simulink model "gm_sampleModel1881_2_sub_sub"  (R2023a)
settings: Solver=VariableStepAuto  StartTime=0.0  StopTime=10.0  RelTol=1e-3
libraries: simulink x2, hdlsllib x2
settings Model: Creator=user1  LastModifiedBy=user1
settings OptimizationCC: BlockReduction=off  ConditionallyExecuteInputs=off
settings DebuggingCC: InheritedTsInSrcMsg=none

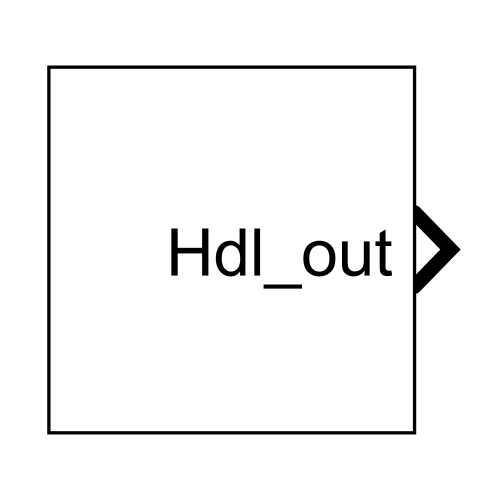
[thumbnail: Simulink's stored preview of the top-level diagram]
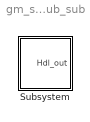
== system gm_sampleModel1881_2_sub_sub ==
  Subsystem : Subsystem

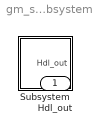
== system gm_sampleModel1881_2_sub_sub/Subsystem ==
  Subsystem : Subsystem
  Hdl_out : Outport  OutDataTypeStr=uint8

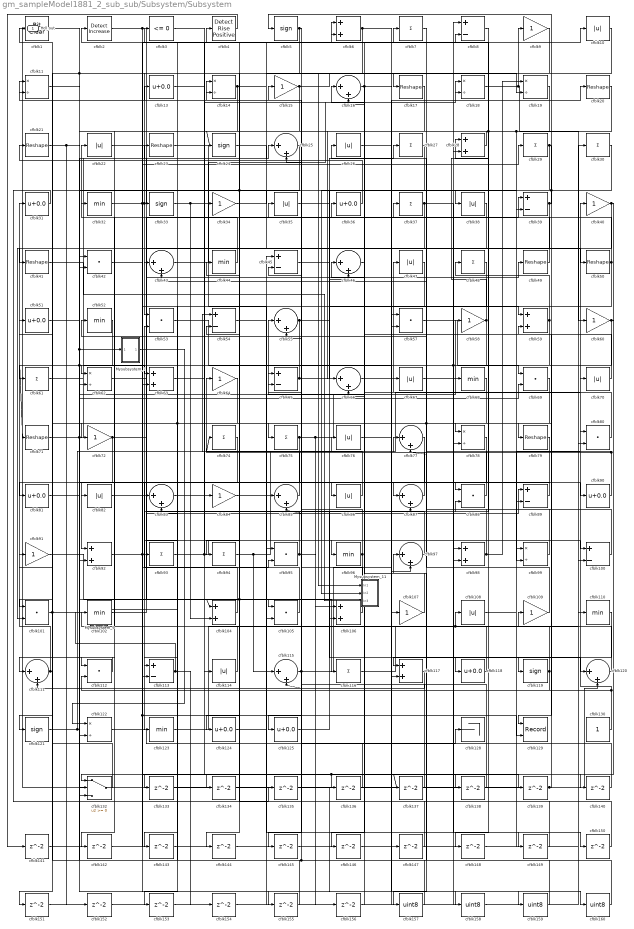
== system gm_sampleModel1881_2_sub_sub/Subsystem/Subsystem ==
  Mysubsystem_11 : Subsystem  TreatAsAtomicUnit=on  RTWFcnName=Mysubsystem_11
      settings: RTWFcnNameOpts=User specified  RTWFileNameOpts=Use function name
  Mysubsystem_7 : Subsystem  TreatAsAtomicUnit=on  RTWFcnName=Mysubsystem_7
      settings: RTWFcnNameOpts=User specified  RTWFileNameOpts=Use function name
  Mysubsystem_9 : Subsystem  TreatAsAtomicUnit=on  RTWFcnName=Mysubsystem_9
      settings: RTWFcnNameOpts=User specified  RTWFileNameOpts=Use function name
  cfblk1 : simulink/Logic and Bit Operations/Bit Clear  iBit=0
      settings: LibrarySourceBlock=|
      | hdlsllib/Logic and Bit
      | Operations/Bit Clear
  cfblk{10,22,26,35,38,47,67,70,76,82,86,108,114} (13 alike) : Abs  OutDataTypeStr=uint8  SaturateOnIntegerOverflow=off
  cfblk{8,39,45,54,65,89,100,113} (8 alike) : Sum  Inputs=+-  OutDataTypeStr=uint8
  cfblk{42,53,57,69,80,88,95,101,105,112} (10 alike) : DotProduct  OutDataTypeStr=uint8
  cfblk{32,44,52,68,96,102,110,123} (8 alike) : MinMax  OutDataTypeStr=uint8
  cfblk{6,28,59,63,92,98,104,106,117} (9 alike) : Sum  OutDataTypeStr=uint8
  cfblk{9,15,34,40,58,60,64,72,84,91,107,109} (12 alike) : Gain  OutDataTypeStr=uint8
  cfblk{11,14,18..19,62,78,99,122} (8 alike) : Product  Inputs=*/  OutDataTypeStr=uint8  RndMeth=Zero  SaturateOnIntegerOverflow=on
  cfblk{16,25,43,46,55,66,77,83,85,87,97,111,115,120} (14 alike) : Sum  Inputs=|++  OutDataTypeStr=uint8
  cfblk{7,27,29..30,37,48,61,74..75,93..94,116} (12 alike) : Sum  Inputs=+  OutDataTypeStr=uint8
  cfblk{13,31,36,51,81,90,118,124..125} (9 alike) : Bias  Bias=0.0  SaturateOnIntegerOverflow=off
  cfblk{5,24,33,119,121} (5 alike) : Signum
  cfblk128 : Terminator
  cfblk129 : Record  FileSettingsInternal="{\"entries\":[{\"content\":{\"excelSettings\":{\"content\":{},\"type\":\"Streamout.ExcelSettings\"}},\"type\":\"Streamout.FileSettingStorage\",\"uuid\":\"\"}],\"packageUris\":[\"http:\\/\\/schema.mathworks.com\\/mf0\\/streamout_blocks\\/R2020a\"],\"version\":\"1.0\"}"  Layout=[1 1]  SignalsInternal="{\"entries\":[{\"content\":{\"signals\":[{\"content\":{\"blockPath\":[],\"dimensions\":[1],\"domain\":\"\",\"lineColor\":\"#a2142f\",\"plots\":[1],\"port\":1,\"signalID\":47170,\"signalName\":\"cfblk29\"},\"type\":\"RecordBlkView.Signal\",\"uuid\":\"\"},{\"content\":{\"blockPath\":[],\"dimensions\":[1],\"domain\":\"\",\"lineColor\":\"#139fff\",\"plots\":[1],\"port\":2,\"signalID\":47173,\"signalName\":\"cfblk42\"},\"type\":\"RecordBlkView.Signal\",\"uuid\":\"\"}]},\"type\":\"RecordBlkView.InputSignals\",\"uuid\":\"\"}],\"packageUris\":[\"http:\\/\\/schema.mathworks.com\\/mf0\\/streamout_blocks\\/R2020a\"],\"version\":\"1.0\"}"  VisualizationBindings="{\"xyplotplugin\":{\"info\":[{\"series\":[{\"bindingParametersList\":[{\"parameter\":\"X-Axis\",\"signalID\":47170,\"signalName\":\"cfblk29\"},{\"parameter\":\"Y-Axis\",\"signalID\":47173,\"signalName\":\"cfblk42\"}],\"seriesID\":24383}],\"subplotID\":1}]}}"  CompatibilityTag=XY  st=-1
  cfblk130 : Constant  OutDataTypeStr=uint8  SampleTime=-1
  cfblk132 : Switch  OutDataTypeStr=uint8  SaturateOnIntegerOverflow=off  InputSameDT=off
  cfblk{133..156} (24 alike) : Delay  SampleTime=1
  cfblk{157..160} (4 alike) : DataTypeConversion  OutDataTypeStr=uint8  SaturateOnIntegerOverflow=off  RndMeth=Floor
  cfblk{17,20..21,23,41,49..50,71,79} (9 alike) : Reshape
  cfblk2 : simulink/Logic and Bit Operations/Detect Increase  vinit=0.0  OutDataTypeStr=uint8
      settings: LibrarySourceBlock=|
      | hdlsllib/Logic and Bit
      | Operations/Detect
      | Increase
  cfblk3 : hdlsllib/Logic and Bit Operations/Compare To Zero  relop=<=  OutDataTypeStr=uint8
  cfblk4 : hdlsllib/Logic and Bit Operations/Detect Rise Positive  vinit=0  OutDataTypeStr=uint8
  Hdl_out : Outport  OutDataTypeStr=uint8
  wires:
  cfblk88/1 -> cfblk26/1
  cfblk71/1 -> cfblk69/2, cfblk25/1
  cfblk93/1 -> cfblk10/1, cfblk96/1
  cfblk82/1 -> cfblk48/1
  cfblk86/1 -> cfblk64/1
  cfblk123/1 -> cfblk109/1
  cfblk28/1 -> cfblk66/1
  cfblk87/1 -> cfblk55/1
  cfblk130/1 -> cfblk15/1, cfblk40/1
  cfblk77/1 -> cfblk92/1
  cfblk121/1 -> cfblk76/1, cfblk54/1
  cfblk79/1 -> cfblk82/1
  cfblk58/1 -> cfblk125/1, cfblk2/1
  cfblk102/1 -> cfblk89/1
  cfblk80/1 -> cfblk35/1
  cfblk111/1 -> cfblk11/1, cfblk31/1
  cfblk110/1 -> cfblk157/1
  cfblk43/1 -> cfblk18/1
  cfblk19/1 -> cfblk24/1, cfblk118/1
  cfblk122/1 -> cfblk128/1
  cfblk37/1 -> cfblk150/1, cfblk94/1
  cfblk50/1 -> cfblk113/2, cfblk36/1
  cfblk57/1 -> cfblk69/1
  cfblk70/1 -> cfblk16/1
  cfblk47/1 -> cfblk75/1
  cfblk67/1 -> cfblk58/1
  cfblk94/1 -> cfblk115/1, cfblk70/1
  cfblk59/1 -> cfblk62/2, cfblk28/1
  cfblk34/1 -> cfblk38/1
  cfblk120/1 -> cfblk6/2, cfblk108/1
  cfblk75/1 -> cfblk133/1, cfblk156/1, cfblk57/2
  cfblk35/1 -> cfblk59/1
  cfblk78/1 -> cfblk123/1
  cfblk23/1 -> cfblk85/1
  cfblk2/1 -> cfblk155/1, cfblk100/1
  cfblk105/1 -> cfblk44/1
  cfblk95/1 -> cfblk106/1, cfblk14/1
  cfblk124/1 -> cfblk45/1
  cfblk39/1 -> cfblk99/2, cfblk5/1
  cfblk108/1 -> cfblk80/1
  cfblk8/1 -> cfblk78/1
  cfblk53/1 -> cfblk107/1
  cfblk62/1 -> cfblk39/1
  cfblk18/1 -> cfblk60/1, cfblk9/1
  cfblk66/1 -> cfblk47/1
  cfblk3/1 -> cfblk34/1
  cfblk63/1 -> cfblk18/2
  cfblk40/1 -> cfblk101/2, cfblk132/1
  cfblk92/1 -> cfblk95/2, cfblk29/1, cfblk49/1
  cfblk5/1 -> cfblk145/1, cfblk144/1
  cfblk36/1 -> cfblk21/1
  cfblk112/1 -> cfblk111/1
  cfblk30/1 -> cfblk106/2, cfblk79/1
  cfblk44/1 -> cfblk22/1
  cfblk118/1 -> cfblk3/1
  cfblk81/1 -> cfblk68/1
  cfblk91/1 -> cfblk105/1
  cfblk55/1 -> cfblk117/2, cfblk92/2, cfblk71/1
  cfblk109/1 -> cfblk67/1
  cfblk85/1 -> cfblk54/2
  cfblk14/1 -> cfblk19/2, cfblk72/1
  cfblk99/1 -> cfblk37/1
  cfblk60/1 -> cfblk140/1, cfblk98/2, cfblk105/2
  cfblk115/1 -> cfblk85/2, cfblk20/1
  cfblk98/1 -> cfblk19/1, cfblk77/1
  cfblk17/1 -> cfblk53/1
  cfblk107/1 -> cfblk46/1
  cfblk96/1 -> cfblk13/1, cfblk134/1, cfblk122/2
  cfblk38/1 -> cfblk121/1
  cfblk10/1 -> cfblk43/1
  cfblk20/1 -> cfblk148/1, cfblk89/2
  cfblk22/1 -> cfblk46/2
  cfblk119/1 -> cfblk112/2, cfblk102/1
  cfblk46/1 -> cfblk6/1
  cfblk49/1 -> cfblk4/1
  cfblk33/1 -> cfblk139/1, cfblk104/2
  cfblk25/1 -> cfblk81/1, cfblk124/1
  cfblk104/1 -> cfblk53/2
  cfblk100/1 -> cfblk52/1
  cfblk13/1 -> cfblk114/1
  cfblk29/1 -> cfblk86/1, cfblk129/1
  cfblk90/1 -> cfblk74/1, cfblk43/2
  cfblk51/1 -> cfblk90/1, Mysubsystem_7/1(In1)
  cfblk61/1 -> cfblk63/1
  cfblk74/1 -> cfblk113/1
  cfblk72/1 -> cfblk151/1, cfblk116/1
  cfblk11/1 -> cfblk132/2
  cfblk114/1 -> cfblk32/1
  cfblk84/1 -> cfblk87/1
  cfblk132/1 -> cfblk91/1
  cfblk97/1 -> cfblk83/1
  cfblk106/1 -> cfblk65/1, cfblk104/1
  cfblk101/1 -> cfblk51/1, cfblk23/1
  cfblk65/1 -> cfblk27/1, cfblk62/1
  cfblk83/1 -> cfblk84/1
  cfblk116/1 -> cfblk30/1
  cfblk15/1 -> cfblk17/1, cfblk132/3
  cfblk69/1 -> cfblk77/2, cfblk112/1, cfblk93/1
  cfblk21/1 -> cfblk152/1, cfblk39/2
  cfblk6/1 -> cfblk138/1, cfblk41/1, cfblk42/2
  cfblk24/1 -> cfblk50/1
  cfblk117/1 -> cfblk111/2
  cfblk7/1 -> cfblk117/1
  cfblk32/1 -> cfblk8/2, cfblk33/1, cfblk7/1
  cfblk42/1 -> cfblk129/2, cfblk137/1, cfblk136/1
  cfblk52/1 -> cfblk61/1
  cfblk89/1 -> cfblk88/1
  cfblk125/1 -> cfblk88/2
  cfblk16/1 -> cfblk146/1, cfblk119/1
  cfblk113/1 -> cfblk154/1, Mysubsystem_9/1(In1)
  cfblk45/1 -> cfblk120/1
  cfblk68/1 -> cfblk101/1
  cfblk133/1 -> cfblk28/2
  cfblk134/1 -> cfblk120/2
  cfblk31/1 -> cfblk135/1
  cfblk136/1 -> cfblk45/2
  cfblk137/1 -> cfblk11/2
  cfblk138/1 -> cfblk55/2
  cfblk139/1 -> Hdl_out/1, cfblk59/2
  cfblk140/1 -> cfblk25/2
  cfblk4/1 -> cfblk141/1
  cfblk141/1 -> cfblk63/2
  cfblk64/1 -> cfblk142/1
  cfblk142/1 -> cfblk98/1
  cfblk48/1 -> cfblk143/1
  cfblk143/1 -> cfblk57/1
  cfblk144/1 -> cfblk97/2
  cfblk145/1 -> cfblk65/2
  cfblk146/1 -> cfblk99/1
  cfblk26/1 -> cfblk147/1
  cfblk147/1 -> cfblk16/2
  cfblk148/1 -> cfblk80/2
  cfblk54/1 -> cfblk149/1
  cfblk149/1 -> cfblk14/2
  cfblk150/1 -> cfblk8/1
  cfblk151/1 -> cfblk95/1
  cfblk152/1 -> cfblk78/2
  cfblk153/1 -> cfblk100/2
  cfblk154/1 -> cfblk87/2
  cfblk155/1 -> cfblk83/2
  cfblk156/1 -> cfblk66/2
  cfblk157/1 -> cfblk42/1, cfblk115/2
  cfblk76/1 -> cfblk158/1
  cfblk158/1 -> cfblk110/1
  cfblk135/1 -> cfblk159/1
  cfblk159/1 -> cfblk1/1
  cfblk1/1 -> cfblk160/1
  cfblk160/1 -> cfblk97/1
  Mysubsystem_7/1(Out1) -> cfblk122/1
  Mysubsystem_9/1(Out1) -> cfblk153/1
  cfblk9/1 -> Mysubsystem_11/1(In1)
  cfblk27/1 -> Mysubsystem_11/2(In2)
  cfblk41/1 -> Mysubsystem_11/3(In3)

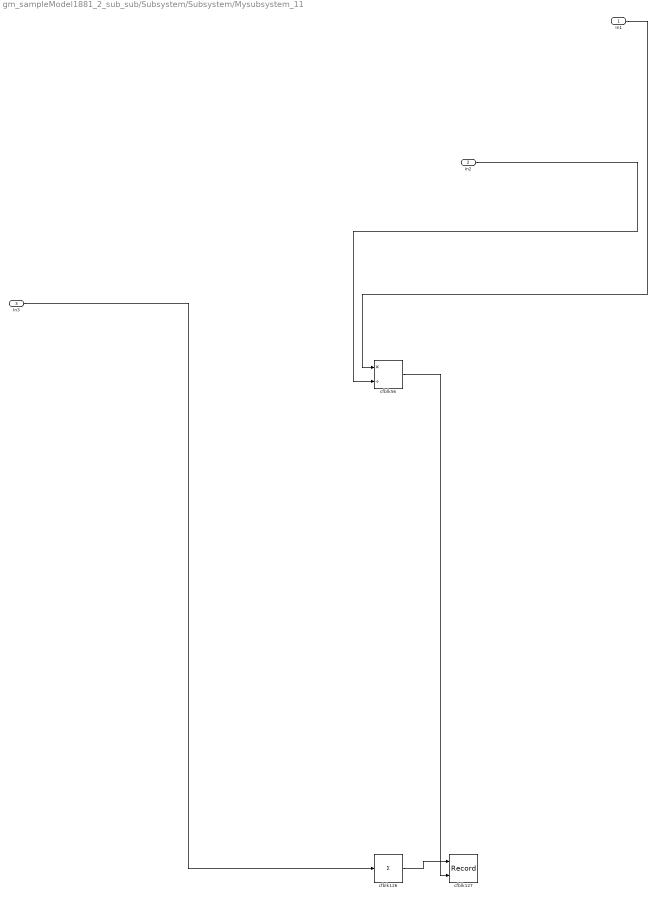
== system gm_sampleModel1881_2_sub_sub/Subsystem/Subsystem/Mysubsystem_11 ==
  In1 : Inport
  In2 : Inport  Port=2
  In3 : Inport  Port=3
  cfblk126 : Sum  Inputs=+
  cfblk127 : Record  FileSettingsInternal="{\"entries\":[{\"content\":{\"excelSettings\":{\"content\":{},\"type\":\"Streamout.ExcelSettings\"}},\"type\":\"Streamout.FileSettingStorage\",\"uuid\":\"\"}],\"packageUris\":[\"http:\\/\\/schema.mathworks.com\\/mf0\\/streamout_blocks\\/R2020a\"],\"version\":\"1.0\"}"  Layout=[1 1]  SignalsInternal="{\"entries\":[{\"content\":{},\"type\":\"RecordBlkView.InputSignals\",\"uuid\":\"\"}],\"packageUris\":[\"http:\\/\\/schema.mathworks.com\\/mf0\\/streamout_blocks\\/R2020a\"],\"version\":\"1.0\"}"  VisualizationBindings="{\"xyplotplugin\":{\"info\":[{\"series\":[],\"subplotID\":1}]}}"  CompatibilityTag=XY  st=-1
  cfblk56 : Product  Inputs=*/  RndMeth=Zero  SaturateOnIntegerOverflow=on
  wires:
  In1/1 -> cfblk56/1
  In2/1 -> cfblk56/2
  cfblk56/1 -> cfblk127/2
  In3/1 -> cfblk126/1
  cfblk126/1 -> cfblk127/1

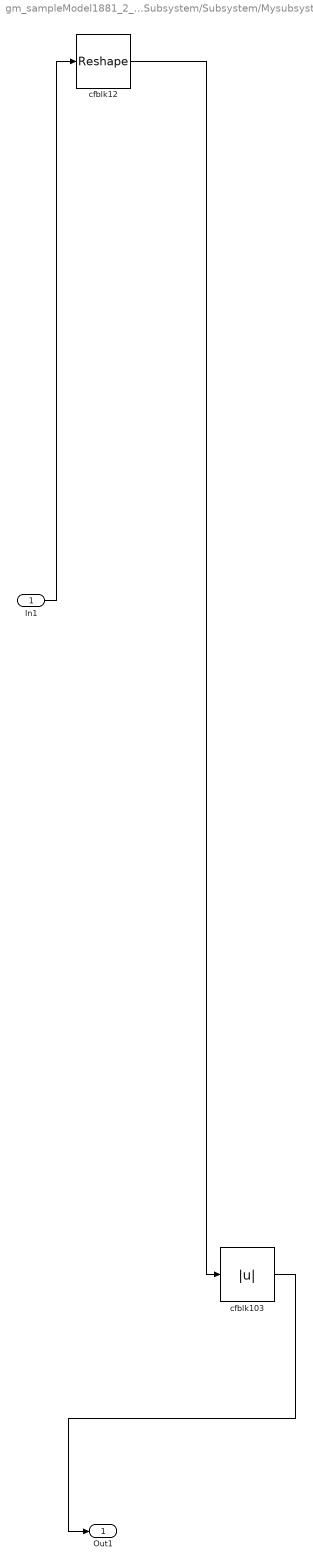
== system gm_sampleModel1881_2_sub_sub/Subsystem/Subsystem/Mysubsystem_7 ==
  In1 : Inport
  cfblk103 : Abs  SaturateOnIntegerOverflow=off
  cfblk12 : Reshape
  Out1 : Outport
  wires:
  cfblk103/1 -> Out1/1
  In1/1 -> cfblk12/1
  cfblk12/1 -> cfblk103/1

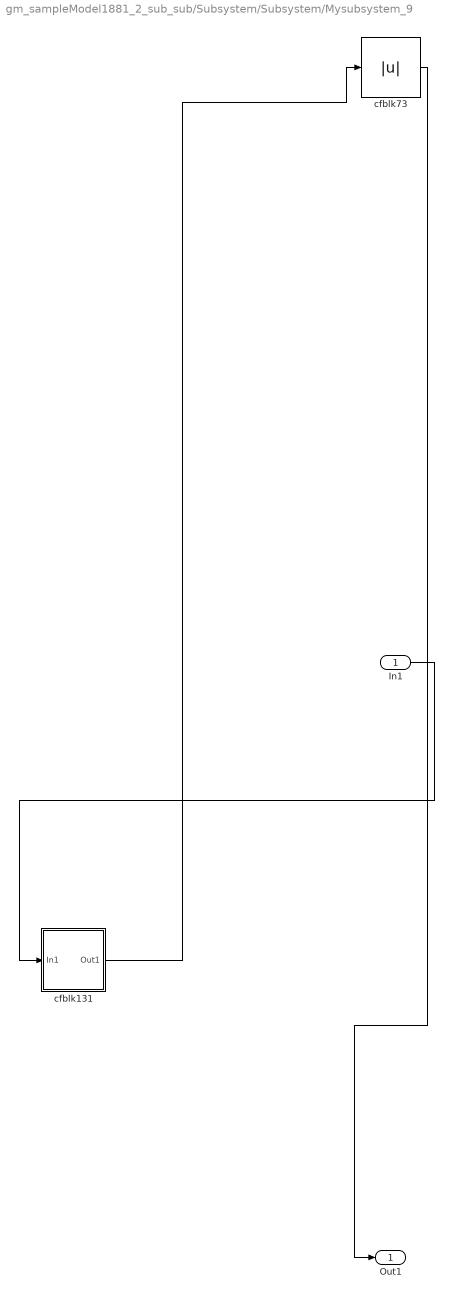
== system gm_sampleModel1881_2_sub_sub/Subsystem/Subsystem/Mysubsystem_9 ==
  In1 : Inport
  cfblk131 : Subsystem
      settings: LibrarySourceBlock=|
      | hdlsllib/Ports &
      | Subsystems/Subsystem
  cfblk73 : Abs  SaturateOnIntegerOverflow=off
  Out1 : Outport
  wires:
  In1/1 -> cfblk131/1(In1)
  cfblk73/1 -> Out1/1
  cfblk131/1(Out1) -> cfblk73/1

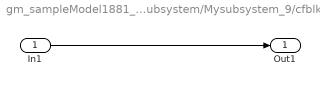
== system gm_sampleModel1881_2_sub_sub/Subsystem/Subsystem/Mysubsystem_9/cfblk131 ==
  In1 : Inport
  Out1 : Outport
  wires:
  In1/1 -> Out1/1
